simulink model "channel"  (Simulink 7.2)
settings: Solver=ode45  StartTime=0.0  StopTime=0.02  RelTol=1e-3
undefined symbols (not defined in the file or in its folder): get
libraries: dspsnks4 x1, commchan3 x1
settings Model: Creator=Administrator  LastModifiedBy=Administrator
settings OptimizationCC: InitFltsAndDblsToZero=on
settings DebuggingCC: SaveWithParameterizedLinksMsg=none  MultiTaskCondExecSysMsg=none
settings RTWCC: IncludeERTFirstTime=on

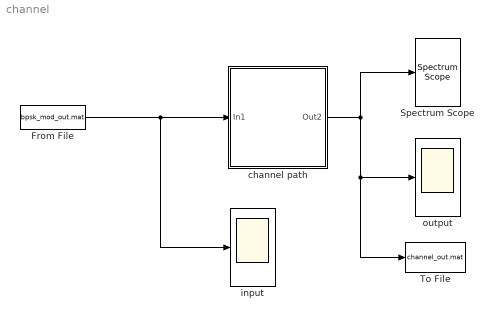
== system channel ==
  From File : FromFile  FileName=bpsk_mod_out.mat  SampleTime=1/5.1e6
  Spectrum Scope : dspsnks4/Spectrum Scope  DialogController=dspdialog.SpectrumScope  DialogControllerArgs=DataTag0  SystemSampleTime=-1  ScopeProperties=on  Domain=Frequency  HorizSpan=1  UseBuffer=on  BufferSize=2048  Overlap=64  inpFftLenInherit=off  FFTlength=128  numAvg=2  DisplayProperties=off  AxisGrid=on  Memory=off  FrameNumber=on  AxisLegend=off  AxisZoom=off  OpenScopeAtSimStart=on  OpenScopeImmediately=off  FigPos=get(0,'defaultfigureposition')  AxisProperties=off  XUnits=Hertz  XRange=[0...Fs/2]  XDisplay=0  InheritXIncr=on  XIncr=1.0  XLabel=Samples  XLimit=Auto  YUnits=dB  XMax=1  XMin=0  YLabel=Magnitude-squared, dB  LineProperties=off  wintypeSpecScope=Hann  RsSpecScope=50  betaSpecScope=5  winsampSpecScope=Periodic
      settings: YMin=-26.8157385137481  YMax=56.6470471111344
  To File : ToFile  Filename=channel_out.mat
  channel path : Subsystem
  input : Scope
      settings: SaveName=ScopeData2
  output : Scope
      settings: TimeRange=0.0002533613445378155  YMin=-30  YMax=40  SaveName=ScopeData3
  wires:
  From File/1 -> channel path/1(In1), input/1
  channel path/1(Out2) -> Spectrum Scope/1, output/1, To File/1

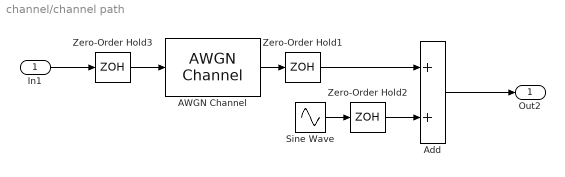
== system channel/channel path ==
  In1 : Inport  OutDataType=sfix(16)  OutScaling=2^0
  AWGN Channel : commchan3/AWGN Channel  SystemSampleTime=-1  seed=67  noiseMode="Signal to noise ratio  (SNR)"  EbNodB=10  EsNodB=10  SNRdB=10  bitsPerSym=1  Ps=1  Tsym=1  variance=1
  Add : Sum  OutDataType=sfix(16)  OutScaling=2^-10
  Sine Wave : Sin  Amplitude=30  Frequency=10.2e5*pi  SampleTime=0
  Zero-Order Hold1 : ZeroOrderHold  SampleTime=1/5.1e6
  Zero-Order Hold2 : ZeroOrderHold  SampleTime=1/5.1e6
  Zero-Order Hold3 : ZeroOrderHold  SampleTime=1/5.1e6
  Out2 : Outport  OutDataType=sfix(16)  OutScaling=2^0
  wires:
  Zero-Order Hold3/1 -> AWGN Channel/1
  In1/1 -> Zero-Order Hold3/1
  Zero-Order Hold2/1 -> Add/2
  Add/1 -> Out2/1
  Zero-Order Hold1/1 -> Add/1
  AWGN Channel/1 -> Zero-Order Hold1/1
  Sine Wave/1 -> Zero-Order Hold2/1
